simulink model "CryoDetXray"  (R2016b)
settings: Solver=ode45  StartTime=0.0  StopTime=10e-5  MaxStep=Tclk/4  RelTol=1e-3
values from neighbouring files (symbols this model uses):
  Fclk = Fadc    (= 307200000)    [setupCryoFPGAxray.m]
  Tclk = 1/Fclk    (= 3.25520833333e-09)    [setupCryoFPGAxray.m]
undefined symbols (not defined in the file or in its folder): AXI4, Lite, lpf, Naxi, xlipgetpartsetting
libraries: xbsIndex_r4 x1091, CryoDetLib x68, simulink x4, hdlsllib x1
(part 5 of 8)

== system CryoDetXray/DspCore/AdcDac 0/Flux Ramp DDC  ==
  note: a burst of 16 outputs
      | every 256 clocks
      |
      | probably want 1 or 2 phi0 every 307.2/256 = 1.2MHz
  note: 16 channel
      | 3rd order
      | decimate by 16
      | CIC LP filter
  note: project out one component of Flux Ramp response
  note: Rotate by input angle
  note: Synchronize
  note: Synchronize frequency error with FluxRamp LO by channel number
      | and digital downconvert
      | mod for 16 channels 22 Sep 2017 SRS
  FreqErrIn : Inport
  FluxRampLO : Inport  Port=2
  AddSub : xbsIndex_r4/AddSub  mode=Addition  use_carryin=off  use_carryout=off  en=off  latency=1  precision=Full  arith_type=Unsigned  n_bits=16  bin_pt=14  quantization=Truncate  overflow=Wrap  use_behavioral_HDL=off  hw_selection=Fabric  pipelined=off  dbl_ovrd=off  block_type=addsub
  Addressable Shift Register : xbsIndex_r4/Addressable Shift Register  infer_latency=off  depth=16  initVector=[0]  en=off  use_behavioral_HDL=off  Optimization=Resource  dbl_ovrd=off  block_type=addrsr
      settings: infoedit="Delay of configurable length.  Any element in the delay line can be addressed and driven onto the output port.<br><br>Hardware notes: Generates fast, compact FIFO-style shift registers or delay lines using SRL16/SRL32 mode of the slice LUTs"
  Addressable Shift Register2 : xbsIndex_r4/Addressable Shift Register  infer_latency=off  depth=16  initVector=[0]  en=off  use_behavioral_HDL=off  Optimization=Resource  dbl_ovrd=off  block_type=addrsr
      settings: infoedit="Delay of configurable length.  Any element in the delay line can be addressed and driven onto the output port.<br><br>Hardware notes: Generates fast, compact FIFO-style shift registers or delay lines using SRL16/SRL32 mode of the slice LUTs"
  Bus Creator : BusCreator  Inputs=3
  Bus Selector : BusSelector  OutputSignals=channel,freqError
  Bus Selector1 : BusSelector  OutputSignals=channel,Qfr,Ifr
  "CIC Compiler 4.0 " : xbsIndex_r4/CIC Compiler 4.0   filter_type=Decimation  number_of_stages=3  differential_delay=1  number_of_channels=16  sample_rate_changes=Fixed  fixed_or_initial_rate=16  minimum_rate=16  maximum_rate=16  ratespecification=Sample_Period  sampleperiod=1  hardwareoversamplingrate=1  quantization=Truncation  output_data_width=20  use_xtreme_dsp_slice=off  use_streaming_interface=off  has_aclken=off  has_aresetn=on  has_dout_tready=off  trim_axipin_name=on  gui_behaviour=Sysgen_GUI  input_data_width=18  ip_name=CIC Compiler  ip_version=4.0  dsptool_ready=true  wrapper_available=true  port_translation_map={ 'aclken' => 'en', 'aresetn' => 'rst' }  ipcore_xco_need_fpga_part=true  ipcore_verbose=false  block_type=cic_compiler_v4_0
  CIC reset1 : Subsystem
  CORDIC 6.0 1 : xbsIndex_r4/CORDIC 6.0   functional_selection=Sin_and_Cos  architectural_configuration=Parallel  pipelining_mode=Optimal  data_format=SignedFraction  phase_format=Scaled_Radians  input_width=16  output_width=16  round_mode=Truncate  iterations=0  precision=0  compensation_scaling=No_Scale_Compensation  coarse_rotation=on  aclken=off  aresetn=off  out_tready=off  cartesian_has_tuser=off  cartesian_has_tlast=off  cartesian_tuser_width=1  phase_has_tuser=off  phase_has_tlast=off  phase_tuser_width=1  out_tlast_behv=Null  flow_control=Blocking  optimize_goal=Resources  trim_axipin_name=on  simulation_type=hybrid_sim  simulation_model=sysgen:cordic_v6_0  data_path_portlist={'s_axis_cartesian_tdata_imag', 's_axis_cartesian_tdata_real', 's_axis_phase_tdata_phase', 'm_axis_dout_tdata_imag', 'm_axis_dout_tdata_real', 'm_axis_dout_tdata_phase','m_axis_dout_tdata'}  ip_name=CORDIC  ip_version=6.0  dsptool_ready=true  ipcore_usecache=true  ipcore_useipmodelcache=true  wrapper_available=true  port_translation_map={ 'aclken' => 'en', 'aresetn' => 'rst' }  block_type=cordic_v6_0
      settings: infoedit=CORDIC 6.0
  Constant : xbsIndex_r4/Constant  const=0  gui_display_data_type=Fixed-point  arith_type=Unsigned  n_bits=4  bin_pt=0  preci_type=Single  exp_width=8  frac_width=24  explicit_period=off  period=1  equ=P=C  opselect=C  inp2=PCIN>>17  opr=+  inp1=P  carry=CIN  dbl_ovrd=off  block_type=constant
  Constant1 : xbsIndex_r4/Constant  const=1  gui_display_data_type=Boolean  arith_type=Boolean  n_bits=4  bin_pt=0  preci_type=Single  exp_width=8  frac_width=24  explicit_period=off  period=1  equ=P=C  opselect=C  inp2=PCIN>>17  opr=+  inp1=P  carry=CIN  dbl_ovrd=off  block_type=constant
  Constant3 : xbsIndex_r4/Constant  const=1  gui_display_data_type=Boolean  arith_type=Boolean  n_bits=4  bin_pt=0  preci_type=Single  exp_width=8  frac_width=24  explicit_period=off  period=1  equ=P=C  opselect=C  inp2=PCIN>>17  opr=+  inp1=P  carry=CIN  dbl_ovrd=off  block_type=constant
  Constant4 : xbsIndex_r4/Constant  const=14  gui_display_data_type=Fixed-point  arith_type=Unsigned  n_bits=4  bin_pt=0  preci_type=Single  exp_width=8  frac_width=24  explicit_period=off  period=1  equ=P=C  opselect=C  inp2=PCIN>>17  opr=+  inp1=P  carry=CIN  dbl_ovrd=off  block_type=constant
  Convert : xbsIndex_r4/Convert  gui_display_data_type=Fixed-point  arith_type="Signed  (2's comp)"  n_bits=16  bin_pt=13  float_type=Single  exp_bits=8  fraction_bits=24  quantization=Truncate  overflow=Wrap  en=off  latency=1  pipeline=off  dbl_ovrd=off  block_type=convert
  Counter : xbsIndex_r4/Counter  cnt_type=Free Running  cnt_to=11  operation=Up  start_count=0  cnt_by_val=1  arith_type=Unsigned  n_bits=4  bin_pt=0  load_pin=off  rst=off  en=on  explicit_period=off  period=50e-9  use_behavioral_HDL=off  implementation=Fabric  dbl_ovrd=off  block_type=counter
  Delay : xbsIndex_r4/Delay  rst=off  infoeditControl=Selection of Reset will increase slice count due to use of real FFs and instead of SRLs  en=off  latency=3  reg_retiming=off  dbl_ovrd=off  block_type=delay
  Delay1 : xbsIndex_r4/Delay  rst=off  infoeditControl=Selection of Reset will increase slice count due to use of real FFs and instead of SRLs  en=off  latency=3  reg_retiming=off  dbl_ovrd=off  block_type=delay
  Delay2 : xbsIndex_r4/Delay  rst=off  infoeditControl=Selection of Reset will increase slice count due to use of real FFs and instead of SRLs  en=off  latency=1  reg_retiming=off  dbl_ovrd=off  block_type=delay
  Delay3 : xbsIndex_r4/Delay  rst=off  infoeditControl=Selection of Reset will increase slice count due to use of real FFs and instead of SRLs  en=off  latency=15  reg_retiming=off  dbl_ovrd=off  block_type=delay
  Delay4 : xbsIndex_r4/Delay  rst=off  infoeditControl=Selection of Reset will increase slice count due to use of real FFs and instead of SRLs  en=off  latency=1  reg_retiming=off  dbl_ovrd=off  block_type=delay
  Delay5 : xbsIndex_r4/Delay  rst=off  infoeditControl=Selection of Reset will increase slice count due to use of real FFs and instead of SRLs  en=off  latency=1  reg_retiming=off  dbl_ovrd=off  block_type=delay
  FR Phase Eror demodulator : Scope  NumInputPorts=4
  Foffset scope1 : Scope  Commented=on  NumInputPorts=8
  Gateway Out{1..2,4,7,9..12,14..16} (11 alike) : xbsIndex_r4/Gateway Out  inherit_from_input=off  hdl_port=off  rows=1  columns=1  UseAsDAC=off  DACChannel='1'  interface=None  automatic_assignment=on  address_offset=hex2dec('00')  intf_name=''  intf_description=''  timing_constraint=None  locs_specified=off  LOCs={}  io_standard={}  block_type=gatewayout
  Gateway Out{3,5..6,8} (4 alike) : xbsIndex_r4/Gateway Out  Commented=on  inherit_from_input=off  hdl_port=off  rows=1  columns=1  UseAsDAC=off  DACChannel='1'  interface=None  automatic_assignment=on  address_offset=hex2dec('00')  intf_name=''  intf_description=''  timing_constraint=None  locs_specified=off  LOCs={}  io_standard={}  block_type=gatewayout
  Logical : xbsIndex_r4/Logical  logical_function=AND  inputs=2  en=off  latency=1  precision=Full  arith_type=Unsigned  n_bits=16  bin_pt=0  align_bp=on  dbl_ovrd=off  block_type=logical
  Logical1 : xbsIndex_r4/Logical  logical_function=OR  inputs=2  en=off  latency=1  precision=Full  arith_type=Unsigned  n_bits=16  bin_pt=0  align_bp=on  dbl_ovrd=off  block_type=logical
  Mult : xbsIndex_r4/Mult  precision=User Defined  arith_type="Signed  (2's comp)"  n_bits=16  bin_pt=15  quantization=Truncate  overflow=Saturate  en=off  latency=3  use_behavioral_HDL=off  opt=Speed  use_embedded=on  optimum_pipeline=off  pipeline=on  dbl_ovrd=off  use_rpm=on  placement_style=Triangular  block_type=mult
  Mult2 : xbsIndex_r4/Mult  precision=User Defined  arith_type="Signed  (2's comp)"  n_bits=16  bin_pt=15  quantization=Truncate  overflow=Saturate  en=off  latency=3  use_behavioral_HDL=off  opt=Speed  use_embedded=on  optimum_pipeline=off  pipeline=on  dbl_ovrd=off  use_rpm=on  placement_style=Triangular  block_type=mult
  Mult3 : xbsIndex_r4/Mult  precision=User Defined  arith_type="Signed  (2's comp)"  n_bits=16  bin_pt=15  quantization=Truncate  overflow=Saturate  en=off  latency=3  use_behavioral_HDL=off  opt=Speed  use_embedded=on  optimum_pipeline=off  pipeline=on  dbl_ovrd=off  use_rpm=on  placement_style=Triangular  block_type=mult
  Mux : Mux  Commented=on  Inputs=2
  Mux1 : Mux  Commented=on  Inputs=2
  Mux2 : xbsIndex_r4/Mux  inputs=2  en=off  latency=1  precision=Full  arith_type=Unsigned  n_bits=16  bin_pt=14  quantization=Truncate  overflow=Wrap  dbl_ovrd=off  block_type=mux
  Phi 0 scope : Scope  Commented=on  NumInputPorts=2
  Relational : xbsIndex_r4/Relational  mode=a=b  op_type=Bool  en=off  latency=1  dbl_ovrd=off  block_type=relational
  Relational1 : xbsIndex_r4/Relational  mode=a!=b  op_type=Bool  en=off  latency=1  dbl_ovrd=off  block_type=relational
  Scale : xbsIndex_r4/Scale  scale_factor=-12  dbl_ovrd=off  block_type=scale
  Out1 : Outport
  wires:
  FreqErrIn/1 -> Bus Selector/1
  FluxRampLO/1 -> Bus Selector1/1
  Addressable Shift Register/1 -> Relational1/2
  Relational/1 -> Logical/1
  Relational1/1 -> Logical/2
  Constant/1 -> Relational1/1, Relational/2
  Logical/1 -> Counter/1
  Bus Selector1/1 -> Delay1/1  "<channel>"
  Counter/1 -> Addressable Shift Register2/2, Addressable Shift Register/2
  Bus Selector/1 -> Delay/1, Relational/1  "<channel>"
  Gateway Out2/1 -> Foffset scope1/1
  Gateway Out4/1 -> Foffset scope1/4
  Gateway Out7/1 -> Foffset scope1/2
  Gateway Out9/1 -> Foffset scope1/5
  Gateway Out10/1 -> Foffset scope1/8
  Gateway Out12/1 -> Foffset scope1/7
  Gateway Out11/1 -> Foffset scope1/6
  Bus Selector/2 -> Gateway Out16/1, Mult/1  "<freqError>"
  Constant4/1 -> CIC reset1/3(N-2)
  [fpgaReset] -> Logical1/1
  [FBreset] -> Logical1/2
  Logical1/1 -> CIC reset1/1(resetIn)
  CIC reset1/1(notResetOut) -> "CIC Compiler 4.0 "/4
  Scale/1 -> Gateway Out1/1, Bus Creator/2  "fluxRampQ"
  Addressable Shift Register2/1 -> Gateway Out14/1, Mult/2
  "CIC Compiler 4.0 "/3 -> Delay5/1
  Mult/1 -> Gateway Out15/1, "CIC Compiler 4.0 "/2
  Constant3/1 -> "CIC Compiler 4.0 "/1
  CIC reset1/2(tlast) -> "CIC Compiler 4.0 "/3
  Delay/1 -> CIC reset1/2(Channel)
  [fluxRampPhaseSetpoint] -> Convert/1
  Constant1/1 -> CORDIC 6.0 1/1
  Delay1/1 -> Delay2/1
  Bus Selector1/2 -> Mult3/1  "<Qfr>"
  Bus Selector1/3 -> Mult2/1  "<Ifr>"
  CORDIC 6.0 1/3 -> Mult3/2, Gateway Out5/1
  CORDIC 6.0 1/4 -> Gateway Out6/1, Mult2/2
  Mult3/1 -> Gateway Out3/1, AddSub/1
  Mult2/1 -> Gateway Out8/1, AddSub/2
  AddSub/1 -> Addressable Shift Register2/1
  "CIC Compiler 4.0 "/1 -> Gateway Out2/1
  "CIC Compiler 4.0 "/2 -> Gateway Out7/1, Mux2/1, Delay4/1  "valid"
  "CIC Compiler 4.0 "/4 -> Gateway Out4/1
  "CIC Compiler 4.0 "/5 -> Gateway Out9/1
  "CIC Compiler 4.0 "/7 -> Gateway Out12/1
  "CIC Compiler 4.0 "/8 -> Gateway Out10/1
  Bus Creator/1 -> Out1/1
  Convert/1 -> CORDIC 6.0 1/2
  Delay2/1 -> Addressable Shift Register/1
  Gateway Out6/1 -> Mux/2
  Gateway Out5/1 -> Mux/1
  Mux/1 -> Phi 0 scope/1
  Gateway Out3/1 -> Mux1/1
  Gateway Out8/1 -> Mux1/2
  Mux1/1 -> Phi 0 scope/2
  Mux2/1 -> Delay3/1, Gateway Out11/1, Bus Creator/1  "channel"
  Delay3/1 -> Mux2/2
  "CIC Compiler 4.0 "/6 -> Mux2/3
  Delay4/1 -> Bus Creator/3  "valid"
  Delay5/1 -> Scale/1
  Gateway Out16/1 -> FR Phase Eror demodulator/1
  Gateway Out14/1 -> FR Phase Eror demodulator/2
  Gateway Out15/1 -> FR Phase Eror demodulator/3
  Gateway Out1/1 -> FR Phase Eror demodulator/4, Foffset scope1/3

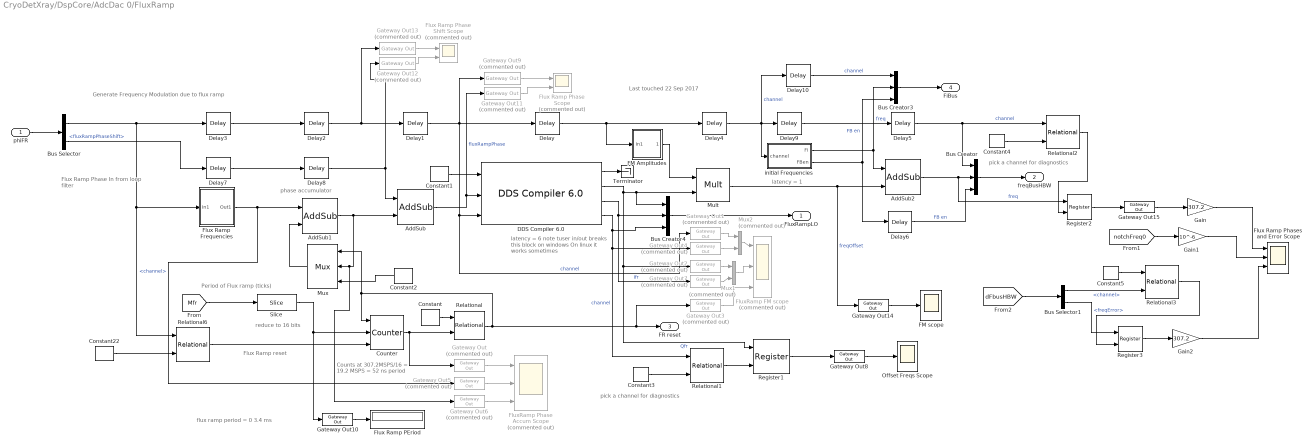
== system CryoDetXray/DspCore/AdcDac 0/FluxRamp ==
  note: latency = 1
  note: flux ramp period = 0 3.4 ms
  note: phase accumulator
  note: Last touched 22 Sep 2017
  note: latency = 6
      | note tuser in/out breaks  this block on windows
      | On linux it works sometimes
  note: Counts at 307.2MSPS/16
      | = 19.2 MSPS
      | = 52 ns period
  note: Flux Ramp reset
  note: Period of Flux ramp (ticks)
  note: Flux Ramp Phase In
      | from loop filter
  note: Generate Frequency Modulation due to flux ramp
  note: reduce to 16 bits
  note: pick a channel for diagnostics
  note: pick a channel for diagnostics
  phiFR : Inport
  AddSub : xbsIndex_r4/AddSub  mode=Addition  use_carryin=off  use_carryout=off  en=off  latency=1  precision=User Defined  arith_type=Unsigned  n_bits=16  bin_pt=16  quantization=Truncate  overflow=Wrap  use_behavioral_HDL=off  hw_selection=Fabric  pipelined=off  dbl_ovrd=off  block_type=addsub
  AddSub1 : xbsIndex_r4/AddSub  mode=Addition  use_carryin=off  use_carryout=off  en=off  latency=3  precision=User Defined  arith_type=Unsigned  n_bits=16  bin_pt=16  quantization=Truncate  overflow=Wrap  use_behavioral_HDL=off  hw_selection=Fabric  pipelined=off  dbl_ovrd=off  block_type=addsub
  AddSub2 : xbsIndex_r4/AddSub  mode=Addition  use_carryin=off  use_carryout=off  en=off  latency=3  precision=User Defined  arith_type=Unsigned  n_bits=24  bin_pt=24  quantization=Truncate  overflow=Saturate  use_behavioral_HDL=on  hw_selection=Fabric  pipelined=off  dbl_ovrd=off  block_type=addsub
  Bus Creator : BusCreator  Inputs=3
  Bus Creator3 : BusCreator  Inputs=3
  Bus Creator4 : BusCreator  Inputs=3
  Bus Selector : BusSelector  OutputSignals=channel,fluxRampPhaseShift
  Bus Selector1 : BusSelector  OutputSignals=channel,freqError
  Constant : xbsIndex_r4/Constant  const=0  gui_display_data_type=Fixed-point  arith_type=Unsigned  n_bits=8  bin_pt=0  preci_type=Single  exp_width=8  frac_width=24  explicit_period=off  period=1  equ=P=C  opselect=C  inp2=PCIN>>17  opr=+  inp1=P  carry=CIN  dbl_ovrd=off  block_type=constant
  Constant1 : xbsIndex_r4/Constant  const=1  gui_display_data_type=Boolean  arith_type=Boolean  n_bits=8  bin_pt=0  preci_type=Single  exp_width=8  frac_width=24  explicit_period=off  period=1  equ=P=C  opselect=C  inp2=PCIN>>17  opr=+  inp1=P  carry=CIN  dbl_ovrd=off  block_type=constant
  Constant2 : xbsIndex_r4/Constant  const=0  gui_display_data_type=Fixed-point  arith_type=Signed (2's comp)  n_bits=16  bin_pt=0  preci_type=Single  exp_width=8  frac_width=24  explicit_period=off  period=1  equ=P=C  opselect=C  inp2=PCIN>>17  opr=+  inp1=P  carry=CIN  dbl_ovrd=off  block_type=constant
  Constant22 : xbsIndex_r4/Constant  const=0  gui_display_data_type=Fixed-point  arith_type=Unsigned  n_bits=8  bin_pt=0  preci_type=Single  exp_width=8  frac_width=24  explicit_period=off  period=1  equ=P=C  opselect=C  inp2=PCIN>>17  opr=+  inp1=P  carry=CIN  dbl_ovrd=off  block_type=constant
  Constant3 : xbsIndex_r4/Constant  const=0  gui_display_data_type=Fixed-point  arith_type=Unsigned  n_bits=4  bin_pt=0  preci_type=Single  exp_width=8  frac_width=24  explicit_period=off  period=1  equ=P=C  opselect=C  inp2=PCIN>>17  opr=+  inp1=P  carry=CIN  dbl_ovrd=off  block_type=constant
  Constant4 : xbsIndex_r4/Constant  const=0  gui_display_data_type=Fixed-point  arith_type=Unsigned  n_bits=4  bin_pt=0  preci_type=Single  exp_width=8  frac_width=24  explicit_period=off  period=1  equ=P=C  opselect=C  inp2=PCIN>>17  opr=+  inp1=P  carry=CIN  dbl_ovrd=off  block_type=constant
  Constant5 : xbsIndex_r4/Constant  const=0  gui_display_data_type=Fixed-point  arith_type=Unsigned  n_bits=4  bin_pt=0  preci_type=Single  exp_width=8  frac_width=24  explicit_period=off  period=1  equ=P=C  opselect=C  inp2=PCIN>>17  opr=+  inp1=P  carry=CIN  dbl_ovrd=off  block_type=constant
  Counter : xbsIndex_r4/Counter  cnt_type=Free Running  cnt_to=Inf  operation=Down  start_count=0  cnt_by_val=1  arith_type=Unsigned  n_bits=16  bin_pt=0  load_pin=on  rst=off  en=on  explicit_period=on  period=Tclk  use_behavioral_HDL=off  implementation=Fabric  dbl_ovrd=off  block_type=counter
  "DDS Compiler 6.0 " : xbsIndex_r4/DDS Compiler 6.0   partspresent=SIN_COS_LUT_only  dds_clock_rate=100  channels=1  mode_of_operation=Standard  modulus=9  parameter_entry=System_Parameters  spurious_free_dynamic_range=45  frequency_resolution=0.4  noise_shaping=None  phase_width=16  output_width=16  output_selection=Sine_and_Cosine  negative_sine=off  negative_cosine=off  amplitude_mode=Unit_Circle  memory_type=Auto  optimization_goal=Auto  dsp48_use=Minimal  resync=off  latency_configuration=Auto  latency=1  has_phase_out=off  has_aclken=off  has_aresetn=off  explicit_period=off  period=1  data_has_tlast=Not_Required  has_tready=off  s_phase_has_tuser=User_Field  m_data_has_tuser=User_Field  m_phase_has_tuser=Not_Required  s_phase_tuser_width=4  output_form=Twos_Complement  s_config_sync_mode=On_Vector  phase_increment=Streaming  output_frequency1=0  output_frequency2=0  output_frequency3=0  output_frequency4=0  output_frequency5=0  output_frequency6=0  output_frequency7=0  output_frequency8=0  output_frequency9=0  output_frequency10=0  output_frequency11=0  output_frequency12=0  output_frequency13=0  output_frequency14=0  output_frequency15=0  output_frequency16=0  pinc1='0'  pinc2='0'  pinc3='0'  pinc4='0'  pinc5='0'  pinc6='0'  pinc7='0'  pinc8='0'  pinc9='0'  pinc10='0'  pinc11='0'  pinc12='0'  pinc13='0'  pinc14='0'  pinc15='0'  pinc16='0'  phase_offset=Streaming  phase_offset_angles1=0  phase_offset_angles2=0  phase_offset_angles3=0  phase_offset_angles4=0  phase_offset_angles5=0  phase_offset_angles6=0  phase_offset_angles7=0  phase_offset_angles8=0  phase_offset_angles9=0  phase_offset_angles10=0  phase_offset_angles11=0  phase_offset_angles12=0  phase_offset_angles13=0  phase_offset_angles14=0  phase_offset_angles15=0  phase_offset_angles16=0  poff1='0'  poff2='0'  poff3='0'  poff4='0'  poff5='0'  poff6='0'  poff7='0'  poff8='0'  poff9='0'  poff10='0'  poff11='0'  poff12='0'  poff13='0'  poff14='0'  poff15='0'  poff16='0'  trim_axipin_name=on  simulation_type=hybrid_sim  simulation_model=sysgen:xddsv6_0_cmodel  data_path_portlist={ 's_axis_config_tdata_poff', 's_axis_config_tdata_chan0_poff', 's_axis_config_tdata_pinc', 's_axis_config_tdata_chan0_pinc', 's_axis_phase_tdata_resync', 's_axis_phase_tdata_chan0_resync', 's_axis_phase_tdata_poff', 's_axis_phase_tdata_chan0_poff', 's_axis_phase_tdata_pinc', 's_axis_phase_tdata_chan0_pinc', 's_axis_phase_tdata_phase_in', 'm_axis_data_tdata_sine', 'm_axis_data_tdata_chan0_sine', 'm_axis_data_tdata_cosine', 'm_axis_data_tdata_chan0_cosine', 'm_axis_phase_tdata_phase_out', 'm_axis_phase_tdata_chan0_phase_out'}  por_mode=false  gui_behaviour=Sysgen  ip_name=DDS Compiler  ip_version=6.0  dsptool_ready=true  wrapper_available=true  port_translation_map={ 'aclken' => 'en', 'aresetn' => 'rst' }  ipcore_usecache=true  ipcore_useipmodelcache=true  ipcore_xco_need_fpga_part=true  ipcore_verbose=false  block_type=dds_compiler_v6_0
  Delay : xbsIndex_r4/Delay  rst=off  infoeditControl=Selection of Reset will increase slice count due to use of real FFs and instead of SRLs  en=off  latency=6  reg_retiming=off  dbl_ovrd=off  block_type=delay
  Delay1 : xbsIndex_r4/Delay  rst=off  infoeditControl=Selection of Reset will increase slice count due to use of real FFs and instead of SRLs  en=off  latency=1  reg_retiming=off  dbl_ovrd=off  block_type=delay
  Delay10 : xbsIndex_r4/Delay  rst=off  infoeditControl=Selection of Reset will increase slice count due to use of real FFs and instead of SRLs  en=off  latency=1  reg_retiming=on  dbl_ovrd=off  block_type=delay
  Delay2 : xbsIndex_r4/Delay  rst=off  infoeditControl=Selection of Reset will increase slice count due to use of real FFs and instead of SRLs  en=off  latency=3  reg_retiming=off  dbl_ovrd=off  block_type=delay
  Delay3 : xbsIndex_r4/Delay  rst=off  infoeditControl=Selection of Reset will increase slice count due to use of real FFs and instead of SRLs  en=off  latency=1  reg_retiming=off  dbl_ovrd=off  block_type=delay
  Delay4 : xbsIndex_r4/Delay  rst=off  infoeditControl=Selection of Reset will increase slice count due to use of real FFs and instead of SRLs  en=off  latency=2  reg_retiming=on  dbl_ovrd=off  block_type=delay
  Delay5 : xbsIndex_r4/Delay  rst=off  infoeditControl=Selection of Reset will increase slice count due to use of real FFs and instead of SRLs  en=off  latency=3  reg_retiming=on  dbl_ovrd=off  block_type=delay
  Delay6 : xbsIndex_r4/Delay  rst=off  infoeditControl=Selection of Reset will increase slice count due to use of real FFs and instead of SRLs  en=off  latency=3  reg_retiming=on  dbl_ovrd=off  block_type=delay
  Delay7 : xbsIndex_r4/Delay  rst=off  infoeditControl=Selection of Reset will increase slice count due to use of real FFs and instead of SRLs  en=off  latency=1  reg_retiming=off  dbl_ovrd=off  block_type=delay
  Delay8 : xbsIndex_r4/Delay  rst=off  infoeditControl=Selection of Reset will increase slice count due to use of real FFs and instead of SRLs  en=off  latency=3  reg_retiming=off  dbl_ovrd=off  block_type=delay
  Delay9 : xbsIndex_r4/Delay  rst=off  infoeditControl=Selection of Reset will increase slice count due to use of real FFs and instead of SRLs  en=off  latency=1  reg_retiming=on  dbl_ovrd=off  block_type=delay
  FM Amplitudes : Subsystem
  FM scope : Scope
  Flux Ramp Frequencies : Subsystem
  Flux Ramp Phase Scope : Scope  Commented=on  NumInputPorts=2
  Flux Ramp Phase Shift Scope : Scope  Commented=on  NumInputPorts=2
  Flux Ramp PEriod : Display
      settings: Decimation=16
  Flux Ramp Phases and Error Scope : Scope  NumInputPorts=3
  FluxRamp Phase Accum Scope : Scope  Commented=on  NumInputPorts=3
  FluxRamp FM scope : Scope  Commented=on  NumInputPorts=3
  Gain : Gain  Gain=307.2
  Gain1 : Gain  Gain=10^-6
  Gain2 : Gain  Gain=307.2
  Gateway Out{,1..7,9,11..13} (12 alike) : xbsIndex_r4/Gateway Out  Commented=on  inherit_from_input=off  hdl_port=off  rows=1  columns=1  UseAsDAC=off  DACChannel='1'  interface=None  automatic_assignment=on  address_offset=hex2dec('00')  intf_name=''  intf_description=''  timing_constraint=None  locs_specified=off  LOCs={}  io_standard={}  block_type=gatewayout
  Gateway Out{8,10,14..15} (4 alike) : xbsIndex_r4/Gateway Out  inherit_from_input=off  hdl_port=off  rows=1  columns=1  UseAsDAC=off  DACChannel='1'  interface=None  automatic_assignment=on  address_offset=hex2dec('00')  intf_name=''  intf_description=''  timing_constraint=None  locs_specified=off  LOCs={}  io_standard={}  block_type=gatewayout
  Mult : xbsIndex_r4/Mult  precision=User Defined  arith_type="Signed  (2's comp)"  n_bits=26  bin_pt=26  quantization=Truncate  overflow=Wrap  en=off  latency=3  use_behavioral_HDL=off  opt=Speed  use_embedded=on  optimum_pipeline=off  pipeline=on  dbl_ovrd=off  use_rpm=on  placement_style=Triangular  block_type=mult
  Mux : xbsIndex_r4/Mux  inputs=2  en=off  latency=13  precision=User Defined  arith_type=Unsigned  n_bits=16  bin_pt=16  quantization=Truncate  overflow=Wrap  dbl_ovrd=off  block_type=mux
  Mux1 : Mux  Commented=on  Inputs=2
  Mux2 : Mux  Commented=on  Inputs=2
  Offset Freqs Scope : Scope
  Register1 : xbsIndex_r4/Register  init=0  rst=off  en=on  dbl_ovrd=off  block_type=register
  Register2 : xbsIndex_r4/Register  init=0  rst=off  en=on  dbl_ovrd=off  block_type=register
  Register3 : xbsIndex_r4/Register  init=0  rst=off  en=on  dbl_ovrd=off  block_type=register
  Relational : xbsIndex_r4/Relational  mode=a=b  op_type=Bool  en=off  latency=1  dbl_ovrd=off  block_type=relational
  Relational{1..3,6} (4 alike) : xbsIndex_r4/Relational  mode=a=b  op_type=Bool  en=off  latency=0  dbl_ovrd=off  block_type=relational
  Slice : xbsIndex_r4/Slice  nbits=16  boolean_output=off  mode=Lower Bit Location + Width  bit1=0  base1=MSB of Input  bit0=0  base0=LSB of Input  dbl_ovrd=off  block_type=slice
  Terminator : Terminator
  initial Frequencies : Subsystem
  FluxRampLO : Outport
  freqBusHBW : Outport  Port=2
  FR reset : Outport  Port=3
  FiBus : Outport  Port=4
  wires:
  Slice/1 -> Gateway Out10/1, Counter/2
  Counter/1 -> Relational/2, Gateway Out/1
  Constant/1 -> Relational/1
  Gateway Out/1 -> FluxRamp Phase Accum Scope/1
  Constant1/1 -> "DDS Compiler 6.0 "/1
  AddSub/1 -> Gateway Out11/1, "DDS Compiler 6.0 "/2  "fluxRampPhase"
  AddSub1/1 -> Gateway Out6/1, Mux/2, AddSub/2
  Constant2/1 -> Mux/3
  Mux/1 -> AddSub1/2
  Relational/1 -> Gateway Out3/1, FR reset/1, Mux/1, Counter/1
  "DDS Compiler 6.0 "/2 -> Register1/1, Gateway Out2/1, Bus Creator4/1, Mult/2  "Qfr"
  Gateway Out3/1 -> FluxRamp FM scope/3
  Constant22/1 -> Relational6/2
  Relational6/1 -> Counter/3
  Mux2/1 -> FluxRamp FM scope/1
  Gateway Out1/1 -> Mux2/1
  Gateway Out4/1 -> Mux2/2
  Delay/1 -> Delay4/1, FM Amplitudes/1(In1)
  Delay3/1 -> Delay2/1
  Delay2/1 -> Delay1/1, Gateway Out13/1
  Delay1/1 -> Gateway Out9/1, Gateway Out1/1, "DDS Compiler 6.0 "/3, Delay/1  "channel"
  Bus Selector/1 -> Relational6/1, Flux Ramp Frequencies/1(In1), Delay3/1  "<channel>"
  FM Amplitudes/1(Out1) -> Mult/1
  AddSub2/1 -> Register2/1, Bus Creator/2  "freq"
  Bus Creator/1 -> freqBusHBW/1
  Mult/1 -> Gateway Out14/1, AddSub2/2  "freqOffset"
  Flux Ramp Frequencies/1(Out1) -> AddSub1/1, Gateway Out5/1
  Bus Selector/2 -> Delay7/1  "<fluxRampPhaseShift>"
  phiFR/1 -> Bus Selector/1
  Delay4/1 -> Delay10/1, Delay9/1, initial Frequencies/1(channel)  "channel"
  initial Frequencies/1(Fi) -> AddSub2/1, Bus Creator3/2  "freq"
  Bus Creator3/1 -> FiBus/1
  [Mfr] -> Slice/1
  "DDS Compiler 6.0 "/1 -> Terminator/1
  Gateway Out5/1 -> FluxRamp Phase Accum Scope/2
  Gateway Out6/1 -> FluxRamp Phase Accum Scope/3
  Gateway Out8/1 -> Offset Freqs Scope/1
  initial Frequencies/2(FBen) -> Delay6/1, Bus Creator3/3  "FB en"
  Delay6/1 -> Bus Creator/3  "FB en"
  Gateway Out10/1 -> Flux Ramp PEriod/1
  Delay7/1 -> Delay8/1
  Delay8/1 -> Gateway Out12/1, AddSub/1
  Constant3/1 -> Relational1/2
  Relational1/1 -> Register1/2
  Register1/1 -> Gateway Out8/1
  "DDS Compiler 6.0 "/4 -> Bus Creator4/3, Relational1/1, Gateway Out4/1  "channel"
  "DDS Compiler 6.0 "/3 -> Gateway Out7/1, Bus Creator4/2  "Ifr"
  Mux1/1 -> FluxRamp FM scope/2
  Gateway Out2/1 -> Mux1/1
  Gateway Out7/1 -> Mux1/2
  Bus Creator4/1 -> FluxRampLO/1
  Gateway Out9/1 -> Flux Ramp Phase Scope/1
  Gateway Out11/1 -> Flux Ramp Phase Scope/2
  Gateway Out13/1 -> Flux Ramp Phase Shift Scope/1
  Gateway Out12/1 -> Flux Ramp Phase Shift Scope/2
  Gateway Out14/1 -> FM scope/1
  Delay9/1 -> Delay5/1
  Delay10/1 -> Bus Creator3/1  "channel"
  Gateway Out15/1 -> Gain/1
  Constant4/1 -> Relational2/2
  Relational2/1 -> Register2/2
  Register2/1 -> Gateway Out15/1
  Delay5/1 -> Bus Creator/1, Relational2/1  "channel"
  Gain/1 -> Flux Ramp Phases and Error Scope/1
  [notchFreq0] -> Gain1/1
  Gain1/1 -> Flux Ramp Phases and Error Scope/2
  [dFbusHBW] -> Bus Selector1/1
  Relational3/1 -> Register3/2
  Bus Selector1/1 -> Relational3/2  "<channel>"
  Constant5/1 -> Relational3/1
  Bus Selector1/2 -> Register3/1  "<freqError>"
  Register3/1 -> Gain2/1
  Gain2/1 -> Flux Ramp Phases and Error Scope/3

== system CryoDetXray/DspCore/AdcDac 0/HBW Sig//Ref LPF ==
  note: High Bandwidth Signal & Reference
      | 3rd order decimate by 8
      | takes 15.4 MSPS down to 1.927 MSPS
  note: Reset Logic
  note: Channel #
  note: Ref
  note: Sig
  In1 : Inport
  Bus Creator : BusCreator  Inputs=2
  Bus Creator1 : BusCreator  Inputs=2
  Bus Selector : BusSelector  OutputSignals=channel,Sig&Ref
  Bus Selector1 : BusSelector  OutputSignals=SignalQ&I,ReferenceQ&I
  Bus Selector2 : BusSelector  OutputSignals=channel,tvalid
  Bus Selector3 : BusSelector  OutputSignals=sigQ,sigI
  Bus Selector4 : BusSelector  OutputSignals=refQ,refI
  CIC Compiler 4.0 {5..6,11..12} (4 alike) : xbsIndex_r4/CIC Compiler 4.0   filter_type=Decimation  number_of_stages=3  differential_delay=1  number_of_channels=16  sample_rate_changes=Fixed  fixed_or_initial_rate=8  minimum_rate=8  maximum_rate=8  ratespecification=Sample_Period  sampleperiod=1  hardwareoversamplingrate=1  quantization=Truncation  output_data_width=24  use_xtreme_dsp_slice=off  use_streaming_interface=off  has_aclken=off  has_aresetn=on  has_dout_tready=off  trim_axipin_name=on  gui_behaviour=Sysgen_GUI  input_data_width=18  ip_name=CIC Compiler  ip_version=4.0  dsptool_ready=true  wrapper_available=true  port_translation_map={ 'aclken' => 'en', 'aresetn' => 'rst' }  ipcore_xco_need_fpga_part=true  ipcore_verbose=false  block_type=cic_compiler_v4_0
  CIC reset : Subsystem
  Constant1 : xbsIndex_r4/Constant  const=1  gui_display_data_type=Boolean  arith_type=Boolean  n_bits=4  bin_pt=0  preci_type=Single  exp_width=8  frac_width=24  explicit_period=off  period=1  equ=P=C  opselect=C  inp2=PCIN>>17  opr=+  inp1=P  carry=CIN  dbl_ovrd=off  block_type=constant
  Constant4 : xbsIndex_r4/Constant  const=14  gui_display_data_type=Fixed-point  arith_type=Unsigned  n_bits=4  bin_pt=0  preci_type=Single  exp_width=8  frac_width=24  explicit_period=off  period=1  equ=P=C  opselect=C  inp2=PCIN>>17  opr=+  inp1=P  carry=CIN  dbl_ovrd=off  block_type=constant
  Display : Display
  Gateway Out{12..18} (7 alike) : xbsIndex_r4/Gateway Out  inherit_from_input=off  hdl_port=off  rows=1  columns=1  UseAsDAC=off  DACChannel='1'  interface=None  automatic_assignment=on  address_offset=hex2dec('00')  intf_name=''  intf_description=''  timing_constraint=None  locs_specified=off  LOCs={}  io_standard={}  block_type=gatewayout
  LPF chan utput : Scope
  Mux : Mux  Inputs=2
  Mux1 : Mux
  Scale{8..11} (4 alike) : xbsIndex_r4/Scale  scale_factor=-9  dbl_ovrd=off  block_type=scale
  Terminator{1..5,14..21,23..24,26..27,49..62} (31 alike) : Terminator
  Out1 : Outport
  wires:
  Bus Selector1/1 -> Bus Selector3/1  "<SignalQ&I>"
  Bus Selector/2 -> Bus Selector1/1  "<Sig&Ref>"
  In1/1 -> Bus Selector/1
  Bus Selector1/2 -> Bus Selector4/1  "<ReferenceQ&I>"
  Constant1/1 -> CIC Compiler 4.0 6/1, CIC Compiler 4.0 5/1, CIC Compiler 4.0 11/1, CIC Compiler 4.0 12/1
  Bus Selector/1 -> Gateway Out15/1, CIC reset/2(Channel)  "<channel>"
  Bus Selector4/1 -> CIC Compiler 4.0 5/2  "<refQ>"
  Bus Selector4/2 -> CIC Compiler 4.0 6/2  "<refI>"
  Mux1/1 -> Bus Creator/2  "I&Qlpf"
  Bus Creator/1 -> Out1/1
  Bus Creator1/1 -> Bus Creator/1, Bus Selector2/1  "channel&tvalid"
  CIC reset/1(notResetOut) -> CIC Compiler 4.0 6/4, CIC Compiler 4.0 5/4, CIC Compiler 4.0 11/4, CIC Compiler 4.0 12/4, Gateway Out18/1
  Constant4/1 -> CIC reset/3(N-2)
  [fpgaReset] -> Gateway Out14/1, CIC reset/1(resetIn)
  CIC reset/2(tlast) -> CIC Compiler 4.0 6/3, CIC Compiler 4.0 5/3, CIC Compiler 4.0 11/3, CIC Compiler 4.0 12/3, Gateway Out17/1
  Gateway Out18/1 -> Terminator5/1
  Gateway Out17/1 -> Terminator4/1
  Gateway Out16/1 -> Terminator3/1
  Gateway Out15/1 -> Terminator2/1
  Gateway Out14/1 -> Terminator1/1
  Bus Selector2/2 -> Gateway Out13/1  "<tvalid>"
  Bus Selector2/1 -> Gateway Out12/1  "<channel>"
  Gateway Out12/1 -> Display/1, Mux/1
  Gateway Out13/1 -> Mux/2
  Mux/1 -> LPF chan utput/1
  CIC Compiler 4.0 5/3 -> Scale8/1
  CIC Compiler 4.0 6/3 -> Scale9/1
  Bus Selector3/2 -> CIC Compiler 4.0 11/2  "<sigI>"
  Bus Selector3/1 -> Gateway Out16/1, CIC Compiler 4.0 12/2  "<sigQ>"
  Scale9/1 -> Mux1/4
  Scale8/1 -> Mux1/3
  CIC Compiler 4.0 11/3 -> Scale10/1
  CIC Compiler 4.0 12/3 -> Scale11/1
  Scale11/1 -> Mux1/1
  Scale10/1 -> Mux1/2
  CIC Compiler 4.0 11/1 -> Terminator14/1
  CIC Compiler 4.0 11/2 -> Terminator15/1
  CIC Compiler 4.0 11/4 -> Terminator16/1
  CIC Compiler 4.0 11/5 -> Terminator17/1
  CIC Compiler 4.0 11/6 -> Terminator18/1
  CIC Compiler 4.0 11/7 -> Terminator19/1
  CIC Compiler 4.0 11/8 -> Terminator20/1
  CIC Compiler 4.0 12/1 -> Terminator21/1
  CIC Compiler 4.0 12/4 -> Terminator23/1
  CIC Compiler 4.0 12/5 -> Terminator24/1
  CIC Compiler 4.0 12/7 -> Terminator26/1
  CIC Compiler 4.0 12/8 -> Terminator27/1
  CIC Compiler 4.0 5/1 -> Terminator49/1
  CIC Compiler 4.0 5/2 -> Terminator50/1
  CIC Compiler 4.0 5/4 -> Terminator51/1
  CIC Compiler 4.0 5/5 -> Terminator52/1
  CIC Compiler 4.0 5/6 -> Terminator53/1
  CIC Compiler 4.0 5/7 -> Terminator54/1
  CIC Compiler 4.0 5/8 -> Terminator55/1
  CIC Compiler 4.0 6/1 -> Terminator56/1
  CIC Compiler 4.0 6/2 -> Terminator57/1
  CIC Compiler 4.0 6/4 -> Terminator58/1
  CIC Compiler 4.0 6/5 -> Terminator59/1
  CIC Compiler 4.0 6/7 -> Terminator60/1
  CIC Compiler 4.0 6/8 -> Terminator61/1
  CIC Compiler 4.0 6/6 -> Terminator62/1
  CIC Compiler 4.0 12/2 -> Bus Creator1/2  "tvalid"
  CIC Compiler 4.0 12/6 -> Bus Creator1/1  "channel"

== system CryoDetXray/DspCore/AdcDac 0/RF switch ==
  note: Enable/disable RF
  note: To DAC
  note: From tone generators
  In1 : Inport
  Assert : xbsIndex_r4/Assert  Commented=on  assert_type=off  type_source=Explicitly  gui_display_data_type=Fixed-point  arith_type="Signed  (2's comp)"  n_bits=16  bin_pt=14  preci_type=Single  exp_width=8  frac_width=24  assert_rate=on  rate_source=Explicitly  period=Tclk  output_port=off  block_type=assert
  Bus Creator : BusCreator  Inputs=4
  Bus Selector : BusSelector  OutputSignals=Q0 sum,I0 sum,Q1 sum,I1 sum
  Constant2 : xbsIndex_r4/Constant  const=0  gui_display_data_type=Fixed-point  arith_type=Signed (2's comp)  n_bits=16  bin_pt=15  preci_type=Single  exp_width=8  frac_width=24  explicit_period=on  period=Tclk  equ=P=C  opselect=C  inp2=PCIN>>17  opr=+  inp1=P  carry=CIN  dbl_ovrd=off  block_type=constant
  Mux{1..4} (4 alike) : xbsIndex_r4/Mux  inputs=2  en=off  latency=1  precision=User Defined  arith_type="Signed  (2's comp)"  n_bits=16  bin_pt=15  quantization=Truncate  overflow=Flag as error  dbl_ovrd=off  block_type=mux
  Out1 : Outport
  wires:
  [RFen] -> Assert/1, Mux4/1, Mux3/1, Mux1/1, Mux2/1
  Constant2/1 -> Mux4/2, Mux3/2, Mux1/2, Mux2/2
  Bus Creator/1 -> Out1/1
  In1/1 -> Bus Selector/1
  Mux2/1 -> Bus Creator/1  "Q0"
  Mux1/1 -> Bus Creator/2  "I0"
  Mux4/1 -> Bus Creator/3  "Q1"
  Mux3/1 -> Bus Creator/4  "I1"
  Bus Selector/1 -> Mux2/3  "<Q0 sum>"
  Bus Selector/2 -> Mux1/3  "<I0 sum>"
  Bus Selector/3 -> Mux4/3  "<Q1 sum>"
  Bus Selector/4 -> Mux3/3  "<I1 sum>"

== system CryoDetXray/DspCore/AdcDac 0/Ref Delay ==
  note: No sideband LO for now,
      | but dummy this to preserce functionality
      | in case we add functionality
  note: Also delay Sideband Local Oscillator I&Q
  note: Delays DAC output data used as Reference for input signal
      | Delay is to compensate for delay of DAC (big), up/downconverter, cable plant, cryostat etc.
      | This is to prevent too much delay mismatch from winding up phase vs. frequency of S21's of sidebands wrt to central line
  In1 : Inport
  Addressable Shift Register{,1..5} (6 alike) : xbsIndex_r4/Addressable Shift Register  infer_latency=on  depth=2  initVector=[0]  en=off  use_behavioral_HDL=on  Optimization=Resource  dbl_ovrd=off  block_type=addrsr
      settings: infoedit="Delay of configurable length.  Any element in the delay line can be addressed and driven onto the output port.<br><br>Hardware notes: Generates fast, compact FIFO-style shift registers or delay lines using SRL16/SRL32 mode of the slice LUTs"
  Bus Creator : BusCreator  Inputs=4
  Bus Selector : BusSelector  OutputSignals=Q0,I0,Q1,I1
  Constant : xbsIndex_r4/Constant  const=0  gui_display_data_type=Fixed-point  arith_type=Signed (2's comp)  n_bits=16  bin_pt=14  preci_type=Single  exp_width=8  frac_width=24  explicit_period=on  period=Tclk  equ=P=C  opselect=C  inp2=PCIN>>17  opr=+  inp1=P  carry=CIN  dbl_ovrd=off  block_type=constant
  Delay{,1..5} (6 alike) : xbsIndex_r4/Delay  rst=off  infoeditControl=Selection of Reset will increase slice count due to use of real FFs and instead of SRLs  en=off  latency=1  reg_retiming=on  dbl_ovrd=off  block_type=delay
  Display : Display
      settings: Decimation=128
  Gateway Out : xbsIndex_r4/Gateway Out  inherit_from_input=off  hdl_port=off  rows=1  columns=1  UseAsDAC=off  DACChannel='1'  interface=None  automatic_assignment=on  address_offset=hex2dec('00')  intf_name=''  intf_description=''  timing_constraint=None  locs_specified=off  LOCs={}  io_standard={}  block_type=gatewayout
  Out1 : Outport
  tag scope: SBIdel=global, SBQdel=global
  wires:
  Addressable Shift Register/1 -> Delay/1  "Q0"
  Addressable Shift Register1/1 -> Delay1/1  "I0"
  In1/1 -> Bus Selector/1
  Bus Selector/2 -> Addressable Shift Register1/1  "<I0>"
  Bus Selector/1 -> Addressable Shift Register/1  "<Q0>"
  Bus Creator/1 -> Out1/1  "refDel"
  Gateway Out/1 -> Display/1
  [SBI] -> Addressable Shift Register2/1
  [SBQ] -> Addressable Shift Register3/1
  [refDel] -> Addressable Shift Register2/2, Addressable Shift Register3/2
  Addressable Shift Register3/1 -> Delay5/1
  Addressable Shift Register2/1 -> Delay4/1
  Constant/1 -> [SBI], [SBQ]
  Addressable Shift Register4/1 -> Delay2/1  "Q1"
  Addressable Shift Register5/1 -> Delay3/1  "I1"
  Bus Selector/4 -> Addressable Shift Register5/1  "<I1>"
  Bus Selector/3 -> Addressable Shift Register4/1  "<Q1>"
  [refDel] -> Addressable Shift Register5/2, Addressable Shift Register4/2, Addressable Shift Register1/2, Addressable Shift Register/2, Gateway Out/1
  Delay4/1 -> [SBIdel]
  Delay5/1 -> [SBQdel]
  Delay/1 -> Bus Creator/1  "Q0"
  Delay1/1 -> Bus Creator/2  "I0"
  Delay2/1 -> Bus Creator/3  "Q1"
  Delay3/1 -> Bus Creator/4  "I1"

== system CryoDetXray/DspCore/AdcDac 0/S21 ==
  note: invalid Op flag set to a constant for now,
      | why is inavlid op not boolean from complex div?
      | comes up NaN which cannot convert to boolean
  note: S21 calculation
      |
      | S21 = Sig/Ref (complex)
  note: Ref
  note: Sig
  In2 : Inport
  Bus Creator : BusCreator  Inputs=3
  Bus Creator1 : BusCreator  Inputs=3
  Bus Selector1 : BusSelector  OutputSignals=channel&tvalid,I&Qlpf
  Complex Divide : Subsystem
  Constant : xbsIndex_r4/Constant  const=1.0  gui_display_data_type=Boolean  arith_type=Boolean  n_bits=16  bin_pt=14  preci_type=Single  exp_width=8  frac_width=24  explicit_period=off  period=1  equ=P=C  opselect=C  inp2=PCIN>>17  opr=+  inp1=P  carry=CIN  dbl_ovrd=off  block_type=constant
  Convert{10..13} (4 alike) : xbsIndex_r4/Convert  gui_display_data_type=Floating-point  arith_type=Floating-point  n_bits=16  bin_pt=14  float_type=Single  exp_bits=8  fraction_bits=24  quantization=Truncate  overflow=Wrap  en=off  latency=2  pipeline=off  dbl_ovrd=off  block_type=convert
  Delay : xbsIndex_r4/Delay  rst=off  infoeditControl=Selection of Reset will increase slice count due to use of real FFs and instead of SRLs  en=off  latency=2  reg_retiming=off  dbl_ovrd=off  block_type=delay
  Delay1 : xbsIndex_r4/Delay  rst=off  infoeditControl=Selection of Reset will increase slice count due to use of real FFs and instead of SRLs  en=off  latency=20  reg_retiming=on  dbl_ovrd=off  block_type=delay
  Delay8 : xbsIndex_r4/Delay  rst=off  infoeditControl=Selection of Reset will increase slice count due to use of real FFs and instead of SRLs  en=off  latency=2  reg_retiming=on  dbl_ovrd=off  block_type=delay
  Demux{1,8,13..16} (6 alike) : Demux  Outputs=2
  Gain : Gain  Gain=1.1
  Gateway Out{1,3..6,15,18..20,35} (10 alike) : xbsIndex_r4/Gateway Out  inherit_from_input=off  hdl_port=off  rows=1  columns=1  UseAsDAC=off  DACChannel='1'  interface=None  automatic_assignment=on  address_offset=hex2dec('00')  intf_name=''  intf_description=''  timing_constraint=None  locs_specified=off  LOCs={}  io_standard={}  block_type=gatewayout
  IIR LPF : Subsystem
  Mux{4..5,9..10} (4 alike) : Mux  Inputs=2
  S21 Input Scope : Scope  NumInputPorts=3
  S21 output Scope : Scope  NumInputPorts=3
  Terminator : Terminator
  S21Bus : Outport
  S21BusLPF : Outport  Port=2
  tag scope: S21Bus=global, S21BusLPF=global
  wires:
  Delay1/1 -> IIR LPF/1(chanIn), Bus Creator/1, Gateway Out15/1  "channel"
  Complex Divide/2(Out_Q) -> IIR LPF/2(Qin), Gateway Out18/1, Bus Creator/2  "etaQ"
  Complex Divide/3(Out_I) -> IIR LPF/3(Iin), Gateway Out19/1, Bus Creator/3  "etaI"
  Bus Creator/1 -> S21Bus/1, [S21Bus]
  Gateway Out6/1 -> Mux5/2
  Gateway Out5/1 -> Mux5/1
  Gateway Out4/1 -> Mux4/2
  Gateway Out3/1 -> Mux4/1
  Mux4/1 -> S21 Input Scope/2
  Mux5/1 -> S21 Input Scope/3
  Demux1/1 -> Gateway Out3/1
  Demux1/2 -> Gateway Out4/1
  Demux8/2 -> Gateway Out6/1
  Demux8/1 -> Gateway Out5/1
  Gateway Out19/1 -> Mux10/2
  Gateway Out18/1 -> Mux10/1
  Mux10/1 -> S21 output Scope/2
  Gateway Out15/1 -> S21 output Scope/1
  Delay/1 -> Delay1/1
  Gateway Out20/1 -> Gain/1
  Gateway Out35/1 -> Mux9/2
  Complex Divide/4(invalid op) -> Gateway Out35/1
  Mux9/1 -> S21 output Scope/3
  Gain/1 -> Mux9/1
  Complex Divide/1(tvalidOut) -> Gateway Out20/1
  Constant/1 -> IIR LPF/4(inavalidIn)
  IIR LPF/3(Iout) -> Bus Creator1/3  "S21I"
  IIR LPF/2(Qout) -> Bus Creator1/2  "S21Q"
  IIR LPF/1(chanOut) -> Bus Creator1/1  "channel"
  Bus Creator1/1 -> S21BusLPF/1, [S21BusLPF]
  Demux13/1 -> Demux1/1, Demux14/1
  Demux13/2 -> Demux8/1, Demux15/1
  Demux15/1 -> Convert12/1
  Demux15/2 -> Convert13/1
  Demux14/2 -> Convert11/1
  Demux14/1 -> Convert10/1
  In2/1 -> Bus Selector1/1
  Demux16/1 -> Delay/1, [ChanIn]  "channel"
  Demux16/2 -> Delay8/1  "tvalid"
  Bus Selector1/1 -> Demux16/1  "<channel&tvalid>"
  Bus Selector1/2 -> Demux13/1  "<I&Qlpf>"
  Convert13/1 -> Complex Divide/6(B_I)
  Convert12/1 -> Complex Divide/5(B_Q)
  Convert11/1 -> Complex Divide/3(A_I)
  Convert10/1 -> Complex Divide/2(A_Q)
  Delay8/1 -> Complex Divide/1(a_tvalid), Complex Divide/4(b_tvalid)
  [ChanIn] -> Terminator/1
  Gateway Out1/1 -> S21 Input Scope/1
  [ChanIn] -> Gateway Out1/1
